simulink model "ctrlauto_tp1_n"  (R2019b)
settings: Solver=ode45  StartTime=0.0  StopTime=6  FixedStep=0.001  RelTol=1e-3
undefined symbols (not defined in the file or in its folder): Ts, ueq, xeq, yref
libraries: cstblocks x1
settings Model: Creator=aghersin  LastModifiedBy=rochi
settings DataIOCC: ReturnWorkspaceOutputs=off
settings DebuggingCC: ArithmeticOperatorsInVariantConditions=warning
settings SFSimCC: SimUseLocalCustomCode=off  CustomCodeUndefinedFunction=UseInterfaceOnly
settings RTWCC: RTWUseLocalCustomCode=off

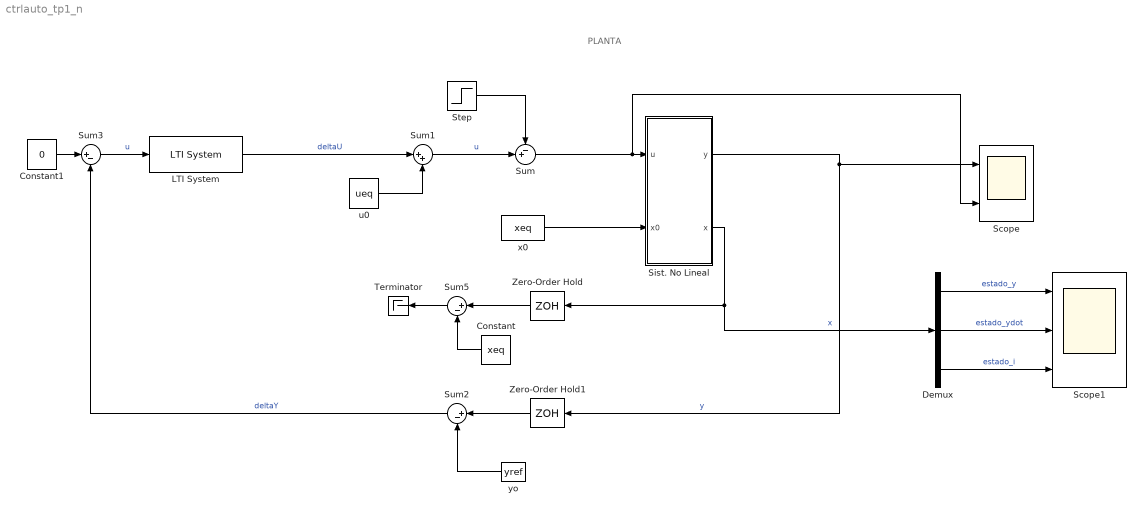
== system ctrlauto_tp1_n ==
  note: PLANTA
  Constant : Constant  Value=xeq
  Constant1 : Constant  Value=0  SampleTime=-1
  Demux : Demux  Outputs=3
  LTI System : cstblocks/LTI System  sys=c_disc  IC=[]
  Scope : Scope  NumInputPorts=2
  Scope1 : Scope  NumInputPorts=3
  "Sist. No Lineal " : Subsystem
  Step : Step  Time=3  After=0.1  SampleTime=0
  Sum : Sum  Inputs=-+|
  Sum1 : Sum  Inputs=|++
  Sum2 : Sum  Inputs=|+-
  Sum3 : Sum  Inputs=|+-
  Sum5 : Sum  Inputs=|+-
  Terminator : Terminator
  Zero-Order Hold : ZeroOrderHold  SampleTime=Ts
  Zero-Order Hold1 : ZeroOrderHold  SampleTime=Ts
  u0 : Constant  Value=ueq
  x0 : Constant  Value=xeq
  yo : Constant  Value=yref
  wires:
  LTI System/1 -> Sum1/1  "deltaU"
  u0/1 -> Sum1/2
  "Sist. No Lineal "/2(x) -> Demux/1, Zero-Order Hold/1  "x"
  "Sist. No Lineal "/1(y) -> Zero-Order Hold1/1, Scope/1  "y"
  x0/1 -> "Sist. No Lineal "/2(x0)
  yo/1 -> Sum2/2
  Constant/1 -> Sum5/2
  Demux/3 -> Scope1/3  "estado_i"
  Demux/2 -> Scope1/2  "estado_ydot"
  Demux/1 -> Scope1/1  "estado_y"
  Sum1/1 -> Sum/2  "u"
  Step/1 -> Sum/1
  Sum/1 -> Scope/2, "Sist. No Lineal "/1(u)
  Zero-Order Hold/1 -> Sum5/1
  Zero-Order Hold1/1 -> Sum2/1
  Sum5/1 -> Terminator/1
  Constant1/1 -> Sum3/1
  Sum2/1 -> Sum3/2  "deltaY"
  Sum3/1 -> LTI System/1  "u"

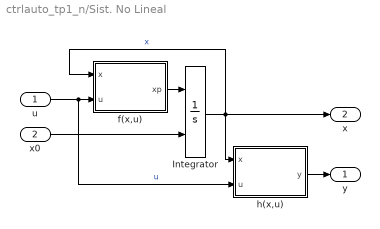
== system ctrlauto_tp1_n/Sist. No Lineal  ==
  u : Inport
  x0 : Inport  Port=2
  Integrator : Integrator  InitialConditionSource=external  ZeroCross=off
  f(x,u) : MATLAB Function  TreatAsAtomicUnit=on
  h(x,u) : MATLAB Function  TreatAsAtomicUnit=on
  y : Outport  VectorParamsAs1DForOutWhenUnconnected=off
  x : Outport  Port=2  VectorParamsAs1DForOutWhenUnconnected=off
  wires:
  h(x,u)/1(y) -> y/1
  u/1 -> h(x,u)/2(u), f(x,u)/2(u)  "u"
  f(x,u)/1(xp) -> Integrator/1
  Integrator/1 -> h(x,u)/1(x), x/1, f(x,u)/1(x)  "x"
  x0/1 -> Integrator/2

== matlab function ctrlauto_tp1_n/Sist. No Lineal /f(x,u) ==
  data: x input; u input; xp output
function xp = f(x,u)

xp1 = x(2);
xp2 = (5*(x(3) + 2)^2)/(2*(x(1) - 1)^2) ...
    - (5*(x(3) - 2)^2)/(2*(x(1) + 1)^2) - 10; 
xp3 = - 4*x(3)^2 + u;

xp = [xp1; xp2; xp3];

== matlab function ctrlauto_tp1_n/Sist. No Lineal /h(x,u) ==
  data: x input; u input; y output
function y = h(x,u)

y=x(1);
